simulink model "etc_logic_callback"  (R2022b)
settings: Solver=VariableStepAuto  StartTime=0.0  StopTime=10.0  RelTol=1e-3  EnableMultiTasking=on
PreLoadFcn:
  | load PI_output.mat
settings Model: Creator=nicholas  LastModifiedBy=bensweet
settings SolverCC: AlgebraicLoopSolver=TrustRegion  AutoInsertRateTranBlk=on
settings DataIOCC: ExternalInput=[PI_output_time, PI_output_data]  LimitDataPoints=on  LoadExternalInput=on  SaveFormat=Array  ReturnWorkspaceOutputs=off  TimeSaveName=tout_blocks  OutputSaveName=yout_blocks
settings OptimizationCC: ExpressionDepthLimit=2147483647  InitFltsAndDblsToZero=on  LifeSpan=1  EfficientTunableParamExpr=on
settings DebuggingCC: UnconnectedInputMsg=warning  UnconnectedOutputMsg=warning  UnconnectedLineMsg=warning  PregeneratedLibrarySubsystemCodeDiagnostic=none  SFMachineParentedDataDiag=warning
settings HardwareCC: ProdBitPerPointer=32  ProdBitPerSizeT=32  ProdBitPerPtrDiffT=32  ProdLargestAtomicFloat=None  ProdIntDivRoundTo=Undefined  ProdEndianess=Unspecified  ProdWordSize=32  ProdHWDeviceType=32-bit Generic
settings ModelReferenceCC: EnableRefExpFcnMdlSchedulingChecks=on  PropagateSignalLabelsOutOfModel=off
settings SFSimCC: SimUseLocalCustomCode=off  MATLABDynamicMemAlloc=off
settings RTWCC: Description=RTW Embedded Coder (no auto configuration)  SystemTargetFile=ert.tlc  GenCodeOnly=on  TemplateMakefile=ert_default_tmf  RTWUseLocalCustomCode=off  DLArmComputeVersion=19.05
settings CodeAppCC: IgnoreCustomStorageClasses=off  CustomSymbolStrType=$N$R$M  StateflowObjectComments=on  InternalIdentifier=Classic
settings ERTTargetCC: TargetFcnLib=ansi_tfl_tmw.mat  MultiwordLength=2048  GenerateSampleERTMain=on  ERTCustomFileTemplate=example_file_process.tlc  ConvertIfToSwitch=off  SuppressUnreachableDefaultCases=off
settings ConfigComp: CovMetricSettings=dw  CovSaveCumulativeToWorkspaceVar=on  CovSaveSingleToWorkspaceVar=on  CovExternalEMLEnable=off  CovSFcnEnable=off

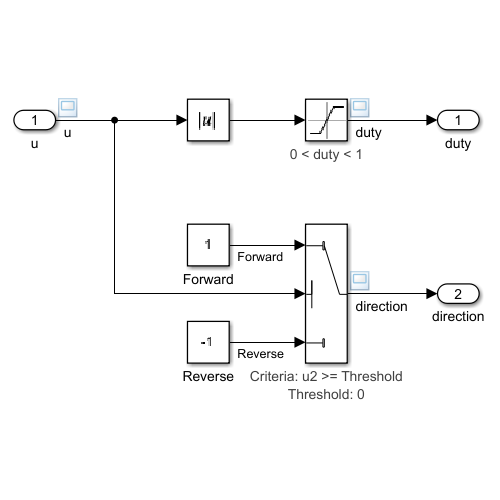
[thumbnail: Simulink's stored preview of the top-level diagram]
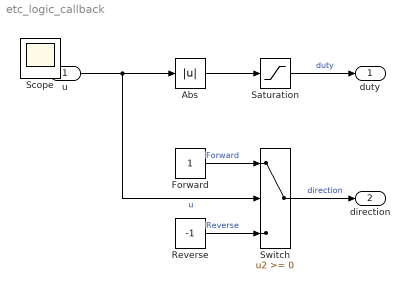
== system etc_logic_callback ==
  u : Inport
  Abs : Abs  SaturateOnIntegerOverflow=off
  Forward : Constant  OutDataTypeStr=double
  Reverse : Constant  Value=-1  OutDataTypeStr=double
  Saturation : Saturate  UpperLimit=1  LowerLimit=0
      settings: AttributesFormatString=%<LowerLimit> < duty < %<UpperLimit>
  Switch : Switch  SaturateOnIntegerOverflow=off  InputSameDT=off
      settings: AttributesFormatString=Criteria: %<Criteria>\nThreshold: %<Threshold>
  duty : Outport  VectorParamsAs1DForOutWhenUnconnected=off
  direction : Outport  Port=2  VectorParamsAs1DForOutWhenUnconnected=off
  Scope : Scope
  wires:
  Abs/1 -> Saturation/1
  Saturation/1 -> duty/1  "duty"
  Switch/1 -> direction/1  "direction"
  Reverse/1 -> Switch/3  "Reverse"
  Forward/1 -> Switch/1  "Forward"
  u/1 -> Switch/2, Abs/1  "u"
